simulink model "Vehicle2DAnimation_Module"  (R2026a)
settings: Solver=VariableStepAuto
settings Model: Creator=MSII  LastModifiedBy=ASUS

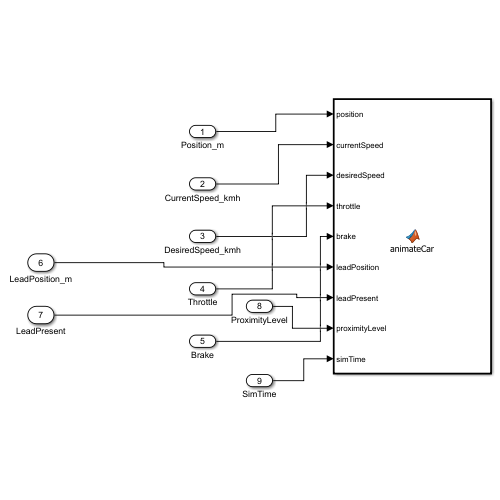
[thumbnail: Simulink's stored preview of the top-level diagram]
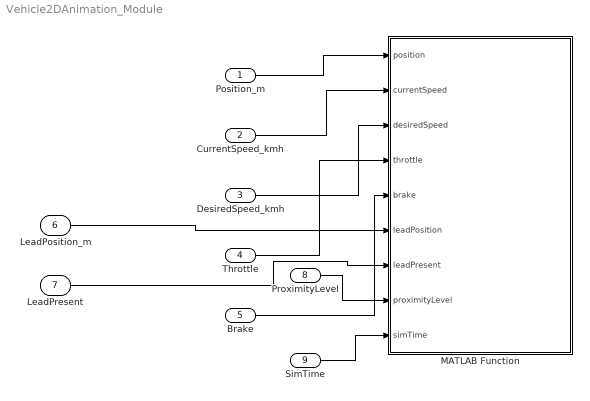
== system Vehicle2DAnimation_Module ==
  "Position_m " : Inport
  "CurrentSpeed_kmh " : Inport  Port=2
  DesiredSpeed_kmh : Inport  Port=3
  Throttle : Inport  Port=4
  Brake : Inport  Port=5
  LeadPosition_m : Inport  Port=6
  LeadPresent : Inport  Port=7  OutDataTypeStr=boolean
  ProximityLevel : Inport  Port=8
  SimTime : Inport  Port=9
  MATLAB Function : MATLAB Function  TreatAsAtomicUnit=on
  wires:
  "Position_m "/1 -> MATLAB Function/1(position)
  "CurrentSpeed_kmh "/1 -> MATLAB Function/2(currentSpeed)
  DesiredSpeed_kmh/1 -> MATLAB Function/3(desiredSpeed)
  Throttle/1 -> MATLAB Function/4(throttle)
  Brake/1 -> MATLAB Function/5(brake)
  LeadPosition_m/1 -> MATLAB Function/6(leadPosition)
  LeadPresent/1 -> MATLAB Function/7(leadPresent)
  ProximityLevel/1 -> MATLAB Function/8(proximityLevel)
  SimTime/1 -> MATLAB Function/9(simTime)

== matlab function Vehicle2DAnimation_Module/MATLAB Function ==
  data: position input; currentSpeed input; desiredSpeed input; throttle input; brake input; leadPosition input; leadPresent input; proximityLevel input; simTime input
function animateCar(position, currentSpeed, desiredSpeed, throttle, brake, leadPosition, leadPresent, proximityLevel, simTime)
%#codegen

coder.extrinsic('updateCar2D');

updateCar2D( ...
    position, ...
    currentSpeed, ...
    desiredSpeed, ...
    throttle, ...
    brake, ...
    leadPosition, ...
    leadPresent, ...
    proximityLevel, ...
    simTime);
end
